simulink model "OHC_NL_Boltzman_Function"  (R2019b)
settings: Solver=VariableStepAuto  StartTime=0.0  StopTime=testtime  RelTol=1e-3
InitFcn:
  | OHC_NL_Boltzman_Test_Parameters
StopFcn:
  | Verify_OHC_NL_Boltzman_Function
undefined symbols (not defined in the file): Fs, s0, s1, shift, x0, x1
libraries: dspsrcs4 x2
settings Model: Creator=mblun  LastModifiedBy=t96f346
settings SFSimCC: CustomCodeUndefinedFunction=UseInterfaceOnly

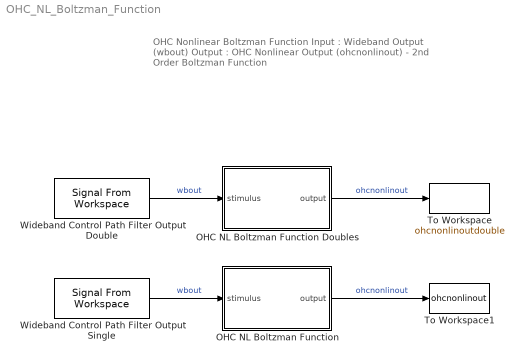
== system OHC_NL_Boltzman_Function ==
  note: OHC Nonlinear Boltzman Function
      |
      | Input : Wideband Output (wbout)
      |
      | Output : OHC Nonlinear Output (ohcnonlinout)
      |
      | - 2nd Order Boltzman Function
  OHC NL Boltzman Function : Subsystem
  OHC NL Boltzman Function Doubles : Subsystem
  To Workspace : ToWorkspace  VariableName=ohcnonlinoutdouble  SampleTime=-1
      settings: Save2DSignal=2-D array (concatenate along first dimension)
  To Workspace1 : ToWorkspace  VariableName=ohcnonlinout  SampleTime=-1
      settings: Save2DSignal=2-D array (concatenate along first dimension)
  Wideband Control Path Filter Output Double : dspsrcs4/Signal From Workspace  X=RxSignalDouble  Ts=1/Fs  nsamps=1  OutputAfterFinalValue=Setting to zero  ignoreOrWarnInputAndFrameLengths=off  OutputFrames=off
  Wideband Control Path Filter Output Single : dspsrcs4/Signal From Workspace  X=RxSignal  Ts=1/Fs  nsamps=1  OutputAfterFinalValue=Setting to zero  ignoreOrWarnInputAndFrameLengths=off  OutputFrames=off
  wires:
  Wideband Control Path Filter Output Double/1 -> OHC NL Boltzman Function Doubles/1(stimulus)  "wbout"
  OHC NL Boltzman Function Doubles/1(output) -> To Workspace/1  "ohcnonlinout"
  OHC NL Boltzman Function/1(output) -> To Workspace1/1  "ohcnonlinout"
  Wideband Control Path Filter Output Single/1 -> OHC NL Boltzman Function/1(stimulus)  "wbout"

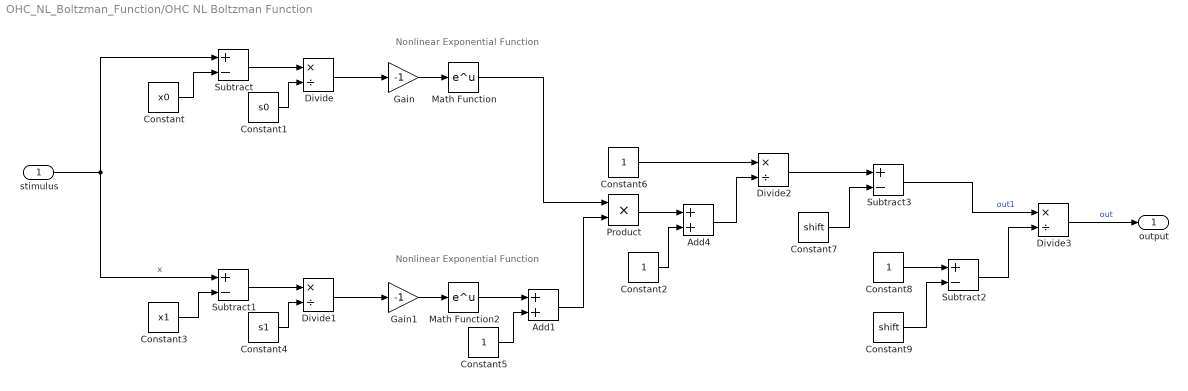
== system OHC_NL_Boltzman_Function/OHC NL Boltzman Function ==
  note: Nonlinear Exponential Function
  note: Nonlinear Exponential Function
  stimulus : Inport
  Add1 : Sum
  Add4 : Sum
  Constant : Constant  Value=x0  OutDataTypeStr=single  SampleTime=-1
  Constant1 : Constant  Value=s0  OutDataTypeStr=single  SampleTime=-1
  Constant{2,5..6,8} (4 alike) : Constant  OutDataTypeStr=single  SampleTime=-1
  Constant3 : Constant  Value=x1  OutDataTypeStr=single  SampleTime=-1
  Constant4 : Constant  Value=s1  OutDataTypeStr=single  SampleTime=-1
  Constant7 : Constant  Value=shift  OutDataTypeStr=single  SampleTime=-1
  Constant9 : Constant  Value=shift  OutDataTypeStr=single  SampleTime=-1
  Divide{,1..3} (4 alike) : Product  Inputs=*/  SaturateOnIntegerOverflow=on  RndMeth=Zero
  Gain : Gain  Gain=-1
  Gain1 : Gain  Gain=-1
  Math Function : Math  SaturateOnIntegerOverflow=on
  Math Function2 : Math  SaturateOnIntegerOverflow=on
  Product : Product
  Subtract{,1..3} (4 alike) : Sum  Inputs=+-
  output : Outport  VectorParamsAs1DForOutWhenUnconnected=off
  wires:
  Constant/1 -> Subtract/2
  stimulus/1 -> Subtract1/1, Subtract/1  "x"
  Subtract/1 -> Divide/1
  Constant1/1 -> Divide/2
  Divide/1 -> Gain/1
  Gain/1 -> Math Function/1
  Constant3/1 -> Subtract1/2
  Subtract1/1 -> Divide1/1
  Constant4/1 -> Divide1/2
  Divide1/1 -> Gain1/1
  Gain1/1 -> Math Function2/1
  Math Function2/1 -> Add1/1
  Constant5/1 -> Add1/2
  Add1/1 -> Product/2
  Constant6/1 -> Divide2/1
  Divide2/1 -> Subtract3/1
  Constant7/1 -> Subtract3/2
  Subtract3/1 -> Divide3/1  "out1"
  Constant8/1 -> Subtract2/1
  Constant9/1 -> Subtract2/2
  Subtract2/1 -> Divide3/2
  Divide3/1 -> output/1  "out"
  Math Function/1 -> Product/1
  Product/1 -> Add4/1
  Constant2/1 -> Add4/2
  Add4/1 -> Divide2/2

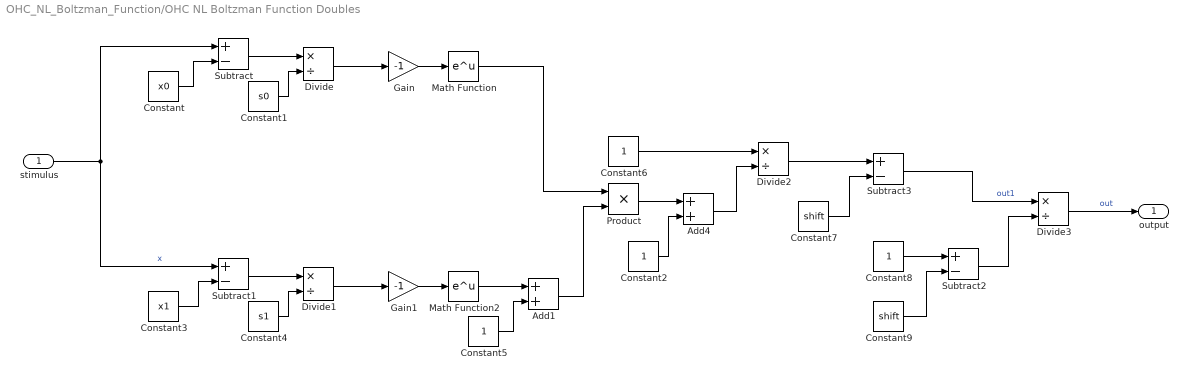
== system OHC_NL_Boltzman_Function/OHC NL Boltzman Function Doubles ==
  stimulus : Inport
  Add1 : Sum
  Add4 : Sum
  Constant : Constant  Value=x0  SampleTime=-1
  Constant1 : Constant  Value=s0  SampleTime=-1
  Constant{2,5..6,8} (4 alike) : Constant  SampleTime=-1
  Constant3 : Constant  Value=x1  SampleTime=-1
  Constant4 : Constant  Value=s1  SampleTime=-1
  Constant7 : Constant  Value=shift  SampleTime=-1
  Constant9 : Constant  Value=shift  SampleTime=-1
  Divide{,1..3} (4 alike) : Product  Inputs=*/  SaturateOnIntegerOverflow=on  RndMeth=Zero
  Gain : Gain  Gain=-1
  Gain1 : Gain  Gain=-1
  Math Function : Math  SaturateOnIntegerOverflow=on
  Math Function2 : Math  SaturateOnIntegerOverflow=on
  Product : Product
  Subtract{,1..3} (4 alike) : Sum  Inputs=+-
  output : Outport  VectorParamsAs1DForOutWhenUnconnected=off
  wires:
  Constant/1 -> Subtract/2
  stimulus/1 -> Subtract1/1, Subtract/1  "x"
  Subtract/1 -> Divide/1
  Constant1/1 -> Divide/2
  Divide/1 -> Gain/1
  Gain/1 -> Math Function/1
  Constant3/1 -> Subtract1/2
  Subtract1/1 -> Divide1/1
  Constant4/1 -> Divide1/2
  Divide1/1 -> Gain1/1
  Gain1/1 -> Math Function2/1
  Math Function2/1 -> Add1/1
  Constant5/1 -> Add1/2
  Add1/1 -> Product/2
  Constant6/1 -> Divide2/1
  Divide2/1 -> Subtract3/1
  Constant7/1 -> Subtract3/2
  Subtract3/1 -> Divide3/1  "out1"
  Constant8/1 -> Subtract2/1
  Constant9/1 -> Subtract2/2
  Subtract2/1 -> Divide3/2
  Divide3/1 -> output/1  "out"
  Math Function/1 -> Product/1
  Product/1 -> Add4/1
  Constant2/1 -> Add4/2
  Add4/1 -> Divide2/2
